simulink library "EcUtilities"  (R2022a)
settings: Solver=VariableStepAuto  StartTime=0.0  StopTime=10.0  RelTol=1e-3

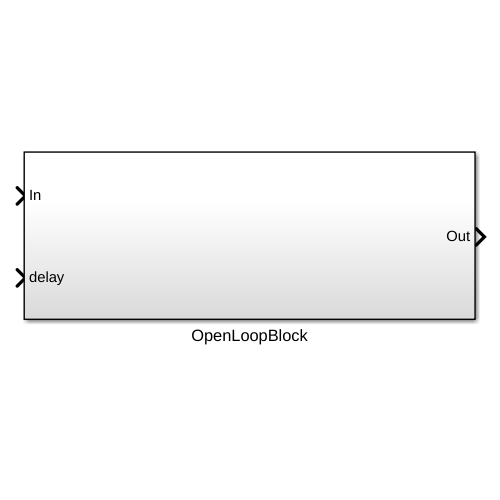
[thumbnail: Simulink's stored preview of the top-level diagram]
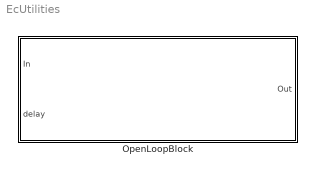
== system EcUtilities ==
  OpenLoopBlock : Subsystem

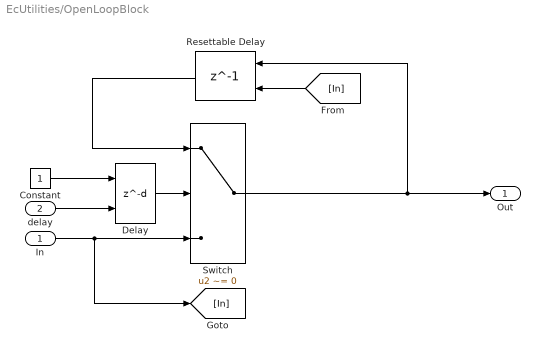
== system EcUtilities/OpenLoopBlock ==
  In : Inport
  delay : Inport  Port=2
  Constant : Constant
  Delay : Delay  DelayLengthSource=Input port  DelayLength=1  InitialCondition=0
  Resettable Delay : Delay  DelayLength=1  InitialConditionSource=Input port
  Switch : Switch  Criteria=u2 ~= 0  SaturateOnIntegerOverflow=off  InputSameDT=off
  Out : Outport
  wires:
  Delay/1 -> Switch/2
  Constant/1 -> Delay/1
  In/1 -> [In], Switch/3
  Switch/1 -> Out/1, Resettable Delay/1
  Resettable Delay/1 -> Switch/1
  [In] -> Resettable Delay/2
  delay/1 -> Delay/2
